simulink model "malha_fechada"  (R2017a)
settings: Solver=VariableStepAuto  StartTime=0.0  StopTime=sampletime  RelTol=1e-3
values from neighbouring files (symbols this model uses):
  C = 200    [Exercicio3.m]    (also in setup.m = 0.0008)
  L = 1/1000    (= 0.001)    [setup.m]
  R = 1    [setup.m]
  Vi = 1    [setup.m]
libraries: simulink x1
settings Model: Creator=05630646761  LastModifiedBy=05630646761

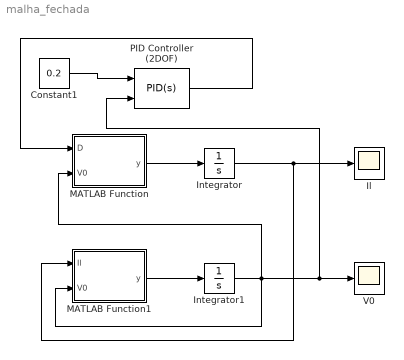
== system malha_fechada ==
  Constant1 : Constant  Value=0.2
  Il : Scope
  Integrator : Integrator
  Integrator1 : Integrator
  MATLAB Function : MATLAB Function  TreatAsAtomicUnit=on
  MATLAB Function1 : MATLAB Function  TreatAsAtomicUnit=on
  PID Controller (2DOF) : simulink/Continuous/PID Controller (2DOF)  Controller=PID  TimeDomain=Continuous-time  SampleTime=-1  IntegratorMethod=Forward Euler  FilterMethod=Forward Euler  Form=Parallel  UseFilter=on  ControllerParametersSource=internal  P=1  I=1  D=0  N=100  b=1  c=1  InitialConditionSource=internal  InitialConditionForIntegrator=0  InitialConditionForFilter=0  ExternalReset=none  LimitOutput=off  UpperSaturationLimit=inf  LowerSaturationLimit=-inf  LinearizeAsGain=on  AntiWindupMode=none  Kb=1  TrackingMode=off  Kt=1  PParamMin=[]  PParamMax=[]  IParamMin=[]  IParamMax=[]  DParamMin=[]  DParamMax=[]  NParamMin=[]  NParamMax=[]  bParamMin=[]  bParamMax=[]  cParamMin=[]  cParamMax=[]  KbParamMin=[]  KbParamMax=[]  KtParamMin=[]  KtParamMax=[]  POutMin=[]  POutMax=[]  IOutMin=[]  IOutMax=[]  DOutMin=[]  DOutMax=[]  NOutMin=[]  NOutMax=[]  bOutMin=[]  bOutMax=[]  cOutMin=[]  cOutMax=[]  KbOutMin=[]  KbOutMax=[]  KtOutMin=[]  KtOutMax=[]  IntegratorOutMin=[]  IntegratorOutMax=[]  FilterOutMin=[]  FilterOutMax=[]  SumOutMin=[]  SumOutMax=[]  Sum1OutMin=[]  Sum1OutMax=[]  Sum2OutMin=[]  Sum2OutMax=[]  Sum3OutMin=[]  Sum3OutMax=[]  SumI1OutMin=[]  SumI1OutMax=[]  SumI2OutMin=[]  SumI2OutMax=[]  SumI3OutMin=[]  SumI3OutMax=[]  SumDOutMin=[]  SumDOutMax=[]  SaturationOutMin=[]  SaturationOutMax=[]  IntegratorContinuousStateAttributes=''  IntegratorStateMustResolveToSignalObject=off  IntegratorRTWStateStorageClass=Auto  FilterContinuousStateAttributes=''  FilterStateMustResolveToSignalObject=off  FilterRTWStateStorageClass=Auto  DifferentiatorICPrevScaledInput=0  DifferentiatorOutMin=[]  DifferentiatorOutMax=[]  InitialConditionSetting=State (most efficient)
  V0 : Scope
  wires:
  MATLAB Function/1(y) -> Integrator/1
  MATLAB Function1/1(y) -> Integrator1/1
  Integrator1/1 -> PID Controller (2DOF)/2, V0/1, MATLAB Function1/2(V0), MATLAB Function/2(V0)
  Integrator/1 -> Il/1, MATLAB Function1/1(Il)
  Constant1/1 -> PID Controller (2DOF)/1
  PID Controller (2DOF)/1 -> MATLAB Function/1(D)

== matlab function malha_fechada/MATLAB Function1 ==
  data: Il input; y output; V0 input; R parameter; C parameter
function y = fcn(Il, V0, R, C)

    y = Il/C - V0/(R*C);

== matlab function malha_fechada/MATLAB Function ==
  data: D input; y output; V0 input; L parameter; Vi parameter
function y = fcn(D, V0, L, Vi)

    y = (D*Vi/L) - V0/L;
